simulink model "multibody_model"  (R2025b)
settings: Solver=ode14x  StartTime=0.0  StopTime=10  FixedStep=0.0001  RelTol=1e-3
settings Model: Creator=leo  LastModifiedBy=leo

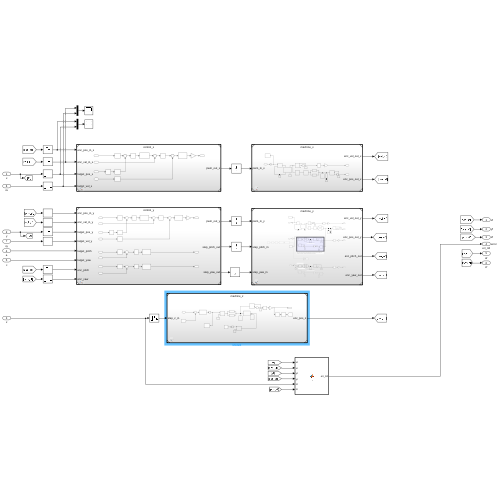
[thumbnail: Simulink's stored preview of the top-level diagram]
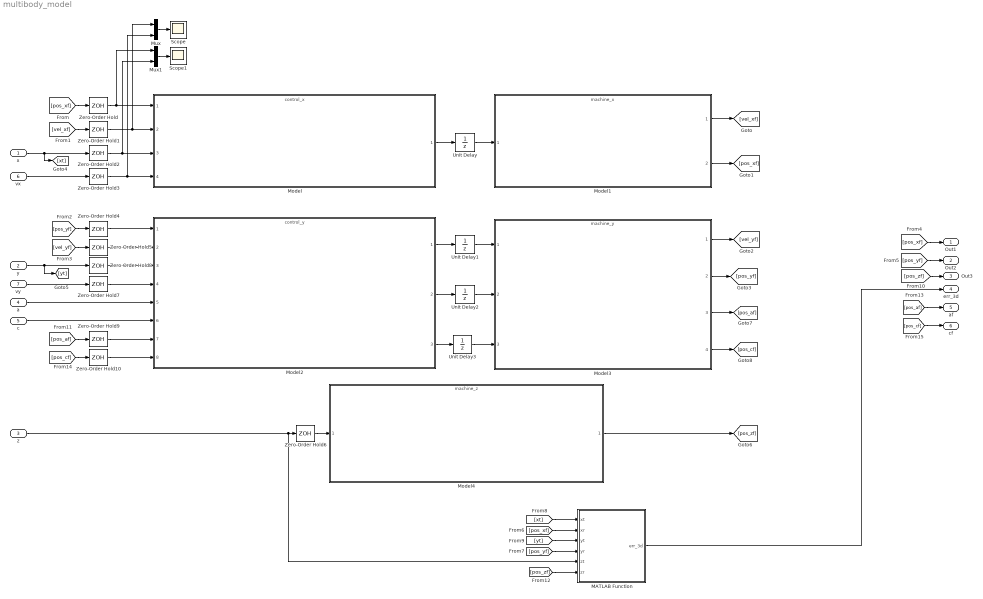
== system multibody_model ==
  x : Inport
  y : Inport  Port=2
  z : Inport  Port=3
  a : Inport  Port=4
  c : Inport  Port=5
  vx : Inport  Port=6
  vy : Inport  Port=7
  MATLAB Function : MATLAB Function  TreatAsAtomicUnit=on
  Model : ModelReference  ModelNameDialog=control_x.slx  SimulationMode=Normal  ModelReferenceVersion=1.36
  Model1 : ModelReference  ModelNameDialog=machine_x.slx  SimulationMode=Normal  ModelReferenceVersion=1.38
  Model2 : ModelReference  ModelNameDialog=control_y.slx  SimulationMode=Normal  ModelReferenceVersion=1.36
  Model3 : ModelReference  ModelNameDialog=machine_y.slx  SimulationMode=Normal  ModelReferenceVersion=1.48
  Model4 : ModelReference  ModelNameDialog=machine_z.slx  SimulationMode=Normal  ModelReferenceVersion=1.37
  Mux : Mux  Inputs=2
  Mux1 : Mux  Inputs=2
  Scope : Scope
      settings: ActiveDisplayYMinimum=-276.36948986064749  ActiveDisplayYMaximum=427.27179530509363
  Scope1 : Scope
      settings: ActiveDisplayYMinimum=0.0059157981462749365  ActiveDisplayYMaximum=0.17745684563436279
  Unit Delay{,1..3} (4 alike) : UnitDelay  SampleTime=0.0001  HasFrameUpgradeWarning=on
  Zero-Order Hold{,2,4,8} (4 alike) : ZeroOrderHold  SampleTime=0.001
  Zero-Order Hold{1,3,5..7,9..10} (7 alike) : ZeroOrderHold  SampleTime=0.0001
  Out1 : Outport  SignalName=xf
  Out2 : Outport  Port=2  SignalName=yf
  Out3 : Outport  Port=3  SignalName=zf
  err_3d : Outport  Port=4  SignalName=error
  af : Outport  Port=5
  cf : Outport  Port=6
  wires:
  Mux/1 -> Scope/1
  Mux1/1 -> Scope1/1
  vx/1 -> Zero-Order Hold3/1
  x/1 -> [xt], Zero-Order Hold2/1
  Model1/1 -> [vel_xf]
  Model1/2 -> [pos_xf]
  [pos_xf] -> Zero-Order Hold/1
  [vel_xf] -> Zero-Order Hold1/1
  Unit Delay/1 -> Model1/1
  Zero-Order Hold/1 -> Model/1, Mux1/1
  Zero-Order Hold1/1 -> Model/2, Mux/1
  Zero-Order Hold2/1 -> Model/3, Mux1/2
  Zero-Order Hold3/1 -> Model/4, Mux/2
  Model2/1 -> Unit Delay1/1
  Unit Delay1/1 -> Model3/1
  Model3/1 -> [vel_yf]
  Model3/2 -> [pos_yf]
  [vel_yf] -> Zero-Order Hold5/1
  Zero-Order Hold5/1 -> Model2/2
  [pos_yf] -> Zero-Order Hold4/1
  Zero-Order Hold4/1 -> Model2/1
  [pos_xf] -> Out1/1
  [pos_yf] -> Out2/1
  c/1 -> Model2/6
  y/1 -> [yt], Zero-Order Hold8/1
  vy/1 -> Zero-Order Hold7/1
  z/1 -> MATLAB Function/5(zt), Zero-Order Hold6/1
  Zero-Order Hold6/1 -> Model4/1
  Zero-Order Hold8/1 -> Model2/3
  Zero-Order Hold7/1 -> Model2/4
  MATLAB Function/1(err_3d) -> err_3d/1
  [pos_xf] -> MATLAB Function/2(xr)
  [pos_yf] -> MATLAB Function/4(yr)
  [xt] -> MATLAB Function/1(xt)
  [yt] -> MATLAB Function/3(yt)
  Model/1 -> Unit Delay/1
  Model2/2 -> Unit Delay2/1
  Unit Delay2/1 -> Model3/2
  Model4/1 -> [pos_zf]
  [pos_zf] -> Out3/1
  Model3/3 -> [pos_af]
  [pos_af] -> Zero-Order Hold9/1
  [pos_zf] -> MATLAB Function/6(zr)
  Zero-Order Hold9/1 -> Model2/7
  a/1 -> Model2/5
  [pos_af] -> af/1
  Model3/4 -> [pos_cf]
  [pos_cf] -> Zero-Order Hold10/1
  Zero-Order Hold10/1 -> Model2/8
  Model2/3 -> Unit Delay3/1
  Unit Delay3/1 -> Model3/3
  [pos_cf] -> cf/1

== matlab function multibody_model/MATLAB Function ==
  data: xt input; err_3d output; xr input; yt input; yr input; zt input; zr input
function err_3d = fcn(xt, xr, yt, yr, zt, zr)
    err_x = xt - xr;
    err_y = yt - yr;
    err_z = zt - zr;
    
    err_3d = sqrt(err_x^2 + err_y^2 + err_z^2);
end
